simulink model "APESHI_LOSS_OF_LOAD"  (R2018a)
settings: Solver=ode45  StartTime=0.0  StopTime=2  RelTol=1e-3  EnableMultiTasking=on
libraries: simulink x1
settings Model: Creator=user  LastModifiedBy=user
settings DataIOCC: LimitDataPoints=on  SaveFormat=Array
settings OptimizationCC: LifeSpan=inf
settings DebuggingCC: SolverPrmCheckMsg=warning  SFUnexpectedBacktrackingDiag=warning  SFNoUnconditionalDefaultTransitionDiag=warning  SFExecutionAtInitializationDiag=none
settings HardwareCC: ProdBitPerPointer=32  ProdBitPerSizeT=32  ProdBitPerPtrDiffT=32  ProdLargestAtomicFloat=None  ProdIntDivRoundTo=Undefined  ProdEndianess=Unspecified  ProdWordSize=32  ProdHWDeviceType=32-bit Generic
settings ModelReferenceCC: PropagateSignalLabelsOutOfModel=off
settings CodeAppCC: StateflowObjectComments=on
settings GRTTargetCC: TargetLangStandard=C89/C90 (ANSI)  GeneratePreprocessorConditionals=Disable all
settings ConfigComp: CovMetricSettings=dw  CovHtmlReporting=on  CovSaveCumulativeToWorkspaceVar=on  CovSaveSingleToWorkspaceVar=on  CovExternalEMLEnable=off  CovSFcnEnable=off

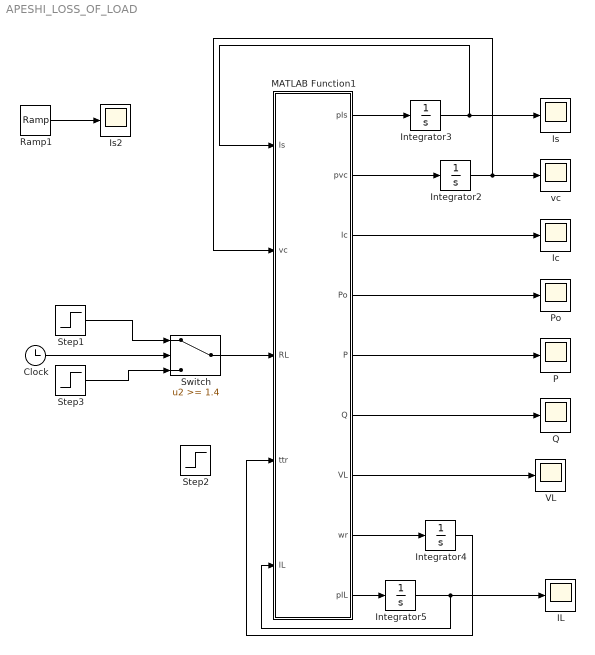
== system APESHI_LOSS_OF_LOAD ==
  Clock : Clock
  IL : Scope
  Ic : Scope
  Integrator2 : Integrator  UpperSaturationLimit=.1  LowerSaturationLimit=-.1
  Integrator3 : Integrator  UpperSaturationLimit=.1  LowerSaturationLimit=-.1
  Integrator4 : Integrator  InitialCondition=0.1  LowerSaturationLimit=-0.1
  Integrator5 : Integrator  AbsoluteTolerance=0.00045  IgnoreLimit=on
  Is : Scope
  Is2 : Scope
  MATLAB Function1 : MATLAB Function  TreatAsAtomicUnit=on
  P : Scope
  Po : Scope
  Q : Scope
  Ramp1 : simulink/Sources/Ramp  slope=-60000  start=0.4  InitialOutput=1000000
  Step1 : Step  Before=2000  After=100000  SampleTime=0.0001
  Step2 : Step  Time=2.5  Before=10e9  After=25  SampleTime=0.0001
  Step3 : Step  Before=100000  After=2000  SampleTime=0.0001
  Switch : Switch  Threshold=1.4  OutMin=5  OutMax=[8]  OutDataTypeStr=double
  VL : Scope
  vc : Scope
  wires:
  MATLAB Function1/2(pvc) -> Integrator2/1
  Integrator2/1 -> vc/1, MATLAB Function1/2(vc)
  MATLAB Function1/8(wr) -> Integrator4/1
  Integrator4/1 -> MATLAB Function1/4(ttr)
  MATLAB Function1/9(pIL) -> Integrator5/1
  Integrator5/1 -> MATLAB Function1/5(IL), IL/1
  MATLAB Function1/3(Ic) -> Ic/1
  MATLAB Function1/4(Po) -> Po/1
  Ramp1/1 -> Is2/1
  MATLAB Function1/7(VL) -> VL/1
  MATLAB Function1/6(Q) -> Q/1
  MATLAB Function1/5(P) -> P/1
  MATLAB Function1/1(pIs) -> Integrator3/1
  Integrator3/1 -> Is/1, MATLAB Function1/1(Is)
  Clock/1 -> Switch/2
  Step1/1 -> Switch/1
  Step3/1 -> Switch/3
  Switch/1 -> MATLAB Function1/3(RL)

== matlab function APESHI_LOSS_OF_LOAD/MATLAB Function1 ==
  data: Is input; vc input; pIs output; pvc output; Ic output; Po output; P output; Q output; VL output; wr output; RL input; ttr input; IL input; pIL output
function [pIs,pvc,Ic,Po,P,Q,VL,wr,pIL] =APESHI(Is,vc,RL,ttr,IL)
 
% performance of Single phase permanent magnet synchronous generator 
% machine parameters
f=50; wr=2*pi*f;xm=0.139;Lmd=0.320;Lmq=0.08; 
L0=(Lmd+Lmq)/2; Ll=(Lmd-Lmq)/2; Ea=2*pi*f*xm*sin(ttr);
C=30*10^-6;Lls=0.067;Rs=27.7;

%single phase self inductance of the machine
Lss=Lls+L0+Ll*cos(2*ttr);
 
% Derivative of the stator current
pIs=inv(Lss)*(Ea-vc+Is*(wr*2*Ll*sin(2*ttr)-Rs));

% The power factor load
pf=0.70;
% the inductive load calculated
LL=(RL/wr)*sqrt(1/pf)^2-1;
% the derivative of load current
pIL=(vc-RL*IL)/LL;
%Load Voltage
VL=RL*IL+(LL*IL);
% The power
Po=vc*Is*pf;
P=vc*IL*pf;
Q=vc*IL*(-pf);
% The stator current
Ic=Is-IL;
% Derivative of capacitor voltage
pvc=(1/C)*Ic;
